simulink model "LQG_plate_ball_controller"  (R2019b)
settings: Solver=FixedStepAuto  StartTime=0.0  StopTime=10.0  RelTol=1e-3
values from neighbouring files (symbols this model uses):
  ballLQRgain = lqr(ballSystem, Q, R)    [LQG_ball.m]    (also in LQG_plate_ball.m; LQR_ball.m)
  I_0 = (3*m_m + m_p)*g/(3*K)    [LQG_plate_ball.m]
  plateLQRgain = lqr(plateSystem, Qp, Rp)    [LQG_plate_ball.m]
  UseUserDefinedBallReference = 1    [LQG_ball.m]    (also in LQG_plate_ball.m; LQR_ball.m; PerformExperiment_CompareModelWithMeasurement.m = 0; Template_PerformExperiment.m = 0)
  UseUserDefinedPlateReference = 1    [LQG_ball.m]    (also in LQG_plate_ball.m; LQR_ball.m; PerformExperiment_CompareModelWithMeasurement.m; Template_PerformExperiment.m = 0)
  Ybop0 = [0.1;0;0;0]    [LQG_ball.m]    (also in LQG_plate_ball.m; LQR_ball.m)
undefined symbols (not defined in the file or in its folder): Continuous, Time
libraries: ctrlSharedLib x2
settings Model: Creator=Duin home  LastModifiedBy=chukh

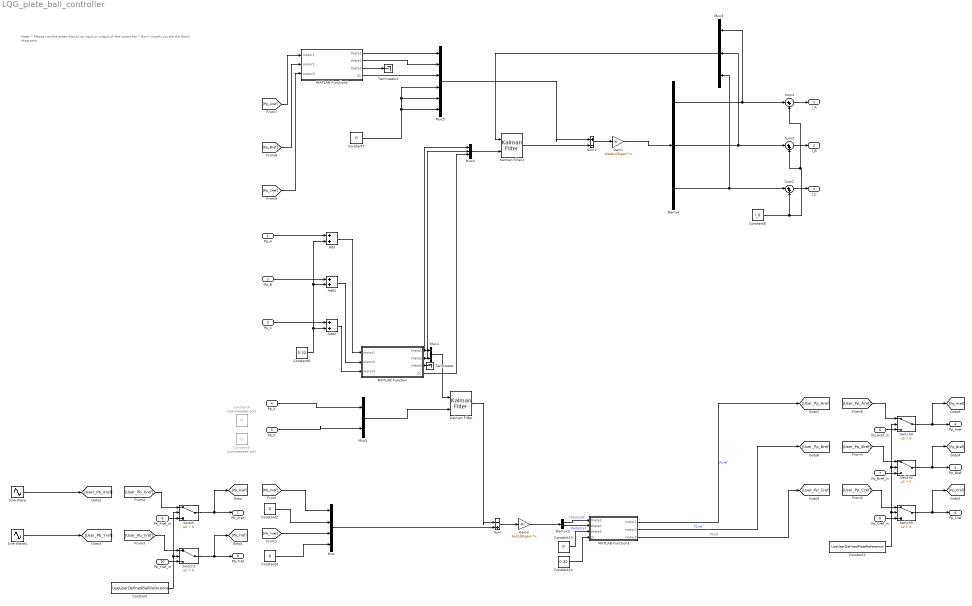
== system LQG_plate_ball_controller ==
  note: Note:
      | * Please use the green blocks as input or output of the controller
      | * Don't modify purple the block diagrams.
  Pp_A : Inport
  Pp_B : Inport  Port=2
  Pp_C : Inport  Port=3
  Pb_X : Inport  Port=4
  Pb_Y : Inport  Port=5
  Pp_Aref_in : Inport  Port=6
  Pp_Bref_in : Inport  Port=7
  Pp_Cref_in : Inport  Port=8
  Pb_Xref_in : Inport  Port=9
  Pb_Yref_in : Inport  Port=10
  Add : Sum
  Add1 : Sum
  Add2 : Sum
  Constant : Constant  Value=UseUserDefinedBallReference
  Constant1 : Constant  Value=UseUserDefinedPlateReference
  Constant{2..3,7,13} (4 alike) : Constant  Value=0
  Constant14 : Constant  Value=0.32
  Constant4 : Constant  Commented=on  Value=0
  Constant5 : Constant  Commented=on  Value=0
  Constant6 : Constant  Value=0.32
  Constant8 : Constant  Value=I_0
  Demux : Demux  Outputs=3
  Demux3 : Demux  Outputs=2
  Gain1 : Gain  Gain=plateLQRgain  Multiplication=Matrix(K*u)
  Gain3 : Gain  Gain=ballLQRgain  Multiplication=Matrix(K*u)
  Kalman Filter : ctrlSharedLib/Kalman Filter  TimeDomain=Continuous-Time  UseCurrentEstimator=on  ModelSource=LTI State-Space Variable  ModelSourceVariable=ballSystem  A=0.95  B=1  C=1  D=0  NumberOfStates=1  NumberOfInputs=1  NumberOfOutputs=1  InitialEstimateSource=Dialog  X0=Ybop0  P0=10  UseK=off  UseGH=off  NumberOfProcessNoiseInputs=1  G=1  TimeInvariantG=on  H=0  TimeInvariantH=on  Q=0.05  TimeInvariantQ=on  R=1  TimeInvariantR=on  N=0  TimeInvariantN=on  AddInputPort=on  AddEnablePort=off  OutputEstimatedY=off  OutputP=off  Ts=-1
      settings: SourceProductBaseCode=CT
  Kalman Filter1 : ctrlSharedLib/Kalman Filter  TimeDomain=Continuous-Time  UseCurrentEstimator=on  ModelSource=LTI State-Space Variable  ModelSourceVariable=plateSystem  A=0.95  B=1  C=1  D=0  NumberOfStates=1  NumberOfInputs=1  NumberOfOutputs=1  InitialEstimateSource=Dialog  X0=[0;0;0.32;0;0;0]  P0=10  UseK=off  UseGH=off  NumberOfProcessNoiseInputs=1  G=1  TimeInvariantG=on  H=0  TimeInvariantH=on  Q=0.05  TimeInvariantQ=on  R=1  TimeInvariantR=on  N=0  TimeInvariantN=on  AddInputPort=on  AddEnablePort=off  OutputEstimatedY=off  OutputP=off  Ts=-1
      settings: SourceProductBaseCode=CT
  MATLAB Function : MATLAB Function  TreatAsAtomicUnit=on
  MATLAB Function1 : MATLAB Function  TreatAsAtomicUnit=on
  MATLAB Function3 : MATLAB Function  TreatAsAtomicUnit=on
  Mux : Mux
  Mux1 : Mux  Inputs=2
  Mux2 : Mux  Inputs=2
  Mux3 : Mux  Inputs=3
  Mux4 : Mux  Inputs=3
  Mux5 : Mux  Inputs=6
  Sine Wave : Sin  Amplitude=0.1  Frequency=pi/5  Phase=pi/2  SampleTime=0
  Sine Wave1 : Sin  Amplitude=0.1  Frequency=pi/5  SampleTime=0
  Sum : Sum  Inputs=|-+
  Sum1 : Sum  Inputs=|+-
  Sum2 : Sum  Inputs=|++
  Sum3 : Sum  Inputs=|++
  Sum4 : Sum  Inputs=|++
  Switch{,1..4} (5 alike) : Switch  Criteria=u2 > Threshold
  Terminator : Terminator
  Terminator2 : Terminator
  I_A : Outport
  I_B : Outport  Port=2
  I_C : Outport  Port=3
  Pp_Aref : Outport  Port=4
  Pp_Bref : Outport  Port=5
  Pp_Cref : Outport  Port=6
  Pb_Xref : Outport  Port=7
  Pb_Yref : Outport  Port=8
  wires:
  Pp_A/1 -> Add/1
  Pp_B/1 -> Add1/1
  Pp_C/1 -> Add2/1
  Pb_X/1 -> Mux2/1
  Pb_Y/1 -> Mux2/2
  Demux/3 -> Sum2/1, Mux3/3
  Demux/2 -> Sum3/1, Mux3/2
  Demux/1 -> Sum4/1, Mux3/1
  Pb_Xref_in/1 -> Switch/3
  Pb_Yref_in/1 -> Switch1/3
  Switch1/1 -> [Pb_Yref], Pb_Yref/1
  Switch/1 -> [Pb_Xref], Pb_Xref/1
  [User_Pb_Xref] -> Switch/1
  [User_Pb_Yref] -> Switch1/1
  Constant/1 -> Switch/2, Switch1/2
  Sine Wave/1 -> [User_Pb_Xref]
  Sine Wave1/1 -> [User_Pb_Yref]
  [Pb_Yref] -> Mux/3
  [Pb_Xref] -> Mux/1
  Pp_Bref_in/1 -> Switch2/3
  [User_Pp_Bref] -> Switch2/1
  Switch3/1 -> [Pp_Cref], Pp_Cref/1
  Switch2/1 -> [Pp_Bref], Pp_Bref/1
  Pp_Cref_in/1 -> Switch3/3
  Constant1/1 -> Switch4/2, Switch2/2, Switch3/2
  [User_Pp_Cref] -> Switch3/1
  [User_Pp_Aref] -> Switch4/1
  Pp_Aref_in/1 -> Switch4/3
  Switch4/1 -> [Pp_Aref], Pp_Aref/1
  [Pp_Aref] -> MATLAB Function1/1(motor1)
  Constant2/1 -> Mux/2
  Constant3/1 -> Mux/4
  MATLAB Function/1(theta1) -> Mux4/1, Mux1/1
  MATLAB Function/2(theta2) -> Mux4/2, Mux1/2
  Mux/1 -> Sum/2
  Gain3/1 -> Demux3/1
  Constant13/1 -> MATLAB Function3/3(theta3)
  MATLAB Function3/2(motor2) -> [User_Pp_Bref]  "P2ref"
  Constant14/1 -> MATLAB Function3/4(Zc)
  Demux3/2 -> MATLAB Function3/2(theta2)  "theta2ref"
  MATLAB Function3/3(motor3) -> [User_Pp_Cref]  "P3ref"
  Demux3/1 -> MATLAB Function3/1(theta1)  "theta1ref"
  MATLAB Function3/1(motor1) -> [User_Pp_Aref]  "P1ref"
  Sum/1 -> Gain3/1
  MATLAB Function/3(theta3) -> Terminator/1
  MATLAB Function/4(Zc) -> Mux4/3
  Mux1/1 -> Kalman Filter/1
  Kalman Filter/1 -> Sum/1
  Mux2/1 -> Kalman Filter/2
  Add/1 -> MATLAB Function/1(motor1)
  Add2/1 -> MATLAB Function/3(motor3)
  Add1/1 -> MATLAB Function/2(motor2)
  Constant6/1 -> Add2/2, Add1/2, Add/2
  Sum1/1 -> Gain1/1
  Mux4/1 -> Kalman Filter1/2
  [Pp_Bref] -> MATLAB Function1/2(motor2)
  [Pp_Cref] -> MATLAB Function1/3(motor3)
  MATLAB Function1/1(theta1) -> Mux5/1
  MATLAB Function1/2(theta2) -> Mux5/2
  MATLAB Function1/4(Zc) -> Mux5/3
  MATLAB Function1/3(theta3) -> Terminator2/1
  Constant7/1 -> Mux5/5, Mux5/4, Mux5/6
  Mux5/1 -> Sum1/1
  Mux3/1 -> Kalman Filter1/1
  Gain1/1 -> Demux/1
  Sum2/1 -> I_C/1
  Sum3/1 -> I_B/1
  Sum4/1 -> I_A/1
  Constant8/1 -> Sum4/2, Sum3/2, Sum2/2
  Kalman Filter1/1 -> Sum1/2

== matlab function LQG_plate_ball_controller/MATLAB Function1 ==
  data: motor1 input; theta1 output; motor2 input; motor3 input; theta2 output; theta3 output; Zc output
% Roll-Pitch-Yaw angles to motors position
% Roll (theta1): rotation about x-axis
% Pitch (theta2): rotation about y-axis
% Yaw (theta3): rotation about z-axis
% See page 12 and Appendix A (Multibody and Nonlinear Dynamics lecture
% notes for further reference
% Motors (1,2,3) -> (A,B,C)

function [theta1,theta2,theta3,Zc] = motorsToAngles2(motor1, motor2, motor3)

%% Define parameters
r = 0.17;
r0B1 = [r; 0; 0];      
r0B2 = [-0.5*r; (sqrt(3)/2)*r; 0];
r0B3 = [-0.5*r; -(sqrt(3)/2)*r; 0];
r0B = [r0B1 r0B2 r0B3];
%r1C1 = r0B1; r1C2 = r0B2; r1C3 = r0B3;
r1C = r0B;

%% Find Zc
Zc = 1/3*(motor1+motor2+motor3);
r0Oc = [0;0;Zc];

%% Assemble matrices
rBC = [0 0 0; 0 0 0; motor1 motor2 motor3];
r0OC = [r0Oc r0Oc r0Oc];

%% Find A10 (Using \ operator to solve a system of linear equation since the matrix r1C is singular)
CPi_rotated = rBC+r0B-r0OC;
P1b = CPi_rotated(:,1);
P2b = CPi_rotated(:,2);
P3b = CPi_rotated(:,3);

%base frame unit vectors
UnitX=[1;0;0];
UnitY=[0;1;0];
UnitZ=[0;0;1];
UnitXp=P1b/sqrt(dot(P1b,P1b));
UnitZp=cross(UnitXp,P3b);
UnitZp=UnitZp/sqrt(dot(UnitZp,UnitZp)); %now length 1
UnitYp=cross(UnitXp,UnitZp);

theta2=asin(-UnitXp(3));
theta3=asin(UnitXp(2)/sqrt(1-UnitXp(3)^2));
theta1=asin(UnitYp(3)/sqrt(1-UnitXp(3)^2));

end

== matlab function LQG_plate_ball_controller/MATLAB Function ==
  data: motor1 input; theta1 output; motor2 input; motor3 input; theta2 output; theta3 output; Zc output
% Roll-Pitch-Yaw angles to motors position
% Roll (theta1): rotation about x-axis
% Pitch (theta2): rotation about y-axis
% Yaw (theta3): rotation about z-axis
% See page 12 and Appendix A (Multibody and Nonlinear Dynamics lecture
% notes for further reference
% Motors (1,2,3) -> (A,B,C)

function [theta1,theta2,theta3,Zc] = motorsToAngles2(motor1, motor2, motor3)

%% Define parameters
r = 0.17;
r0B1 = [r; 0; 0];      
r0B2 = [-0.5*r; (sqrt(3)/2)*r; 0];
r0B3 = [-0.5*r; -(sqrt(3)/2)*r; 0];
r0B = [r0B1 r0B2 r0B3];
%r1C1 = r0B1; r1C2 = r0B2; r1C3 = r0B3;
r1C = r0B;

%% Find Zc
Zc = 1/3*(motor1+motor2+motor3);
r0Oc = [0;0;Zc];

%% Assemble matrices
rBC = [0 0 0; 0 0 0; motor1 motor2 motor3];
r0OC = [r0Oc r0Oc r0Oc];

%% Find A10 (Using \ operator to solve a system of linear equation since the matrix r1C is singular)
CPi_rotated = rBC+r0B-r0OC;
P1b = CPi_rotated(:,1);
P2b = CPi_rotated(:,2);
P3b = CPi_rotated(:,3);

%base frame unit vectors
UnitX=[1;0;0];
UnitY=[0;1;0];
UnitZ=[0;0;1];
UnitXp=P1b/sqrt(dot(P1b,P1b));
UnitZp=cross(UnitXp,P3b);
UnitZp=UnitZp/sqrt(dot(UnitZp,UnitZp)); %now length 1
UnitYp=cross(UnitXp,UnitZp);

theta2=asin(-UnitXp(3));
theta3=asin(UnitXp(2)/sqrt(1-UnitXp(3)^2));
theta1=asin(UnitYp(3)/sqrt(1-UnitXp(3)^2));

end

== matlab function LQG_plate_ball_controller/MATLAB Function3 ==
  data: theta1 input; motor1 output; theta2 input; theta3 input; Zc input; motor2 output; motor3 output
% Roll-Pitch-Yaw angles to motors position
% Roll (theta1): rotation about x-axis
% Pitch (theta2): rotation about y-axis
% Yaw (theta3): rotation about z-axis
% See page 12 and Appendix A (Multibody and Nonlinear Dynamics lecture
% notes for further reference
% Motors (1,2,3) -> (A,B,C)

function [motor1, motor2, motor3] = anglesToMotors(theta1,theta2,theta3,Zc)

%% Define parameters
r = 0.17;
r0B1 = [r; 0; 0];      
r0B2 = [-0.5*r; (sqrt(3)/2)*r; 0];
r0B3 = [-0.5*r; -(sqrt(3)/2)*r; 0];
r0B = [r0B1 r0B2 r0B3];
%r1C1 = r0B1; r1C2 = r0B2; r1C3 = r0B3;
r1C = r0B;
r0Oc = [0;0;Zc];

% Find cos and sin to accelerate calculations
C1 = cos(theta1);S1 = sin(theta1);C2 = cos(theta2);S2 = sin(theta2);C3 = cos(theta3);S3 = sin(theta3);

% Rotation matrices
RotZ = [C3 S3 0; -S3 C3 0; 0 0 1];
RotY = [C2 0 -S2; 0 1 0; S2 0 C2];
RotX = [1 0 0; 0 C1 S1; 0 -S1 C1];

A10 = RotX*RotY*RotZ; A01 = A10';

% Find rCiBi (Vectors representing the motors)
rCiBi = zeros(3,3);
for i=1:3
    rCiBi(:,i) = r0Oc + A01*r1C(:,i) - r0B(:,i);
end

% Outputs to motor are the lengths of the vectors
motor1 = norm(rCiBi(:,1));
motor2 = norm(rCiBi(:,2));
motor3 = norm(rCiBi(:,3));
end
